simulink model "PMSM_Mathematical_Modeling"  (R2022a)
settings: Solver=VariableStepAuto  StartTime=0.0  StopTime=1  RelTol=1e-3
settings Model: Creator=nikos  LastModifiedBy=nikos

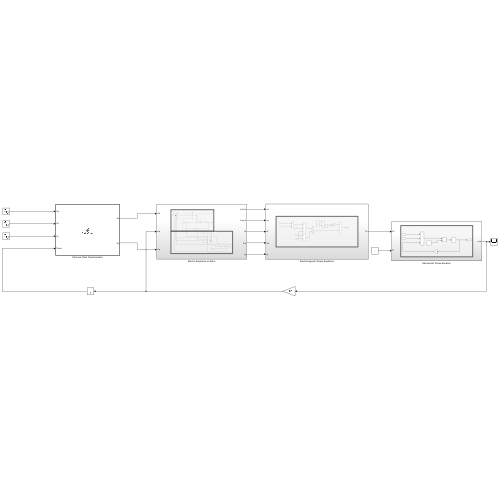
[thumbnail: Simulink's stored preview of the top-level diagram]
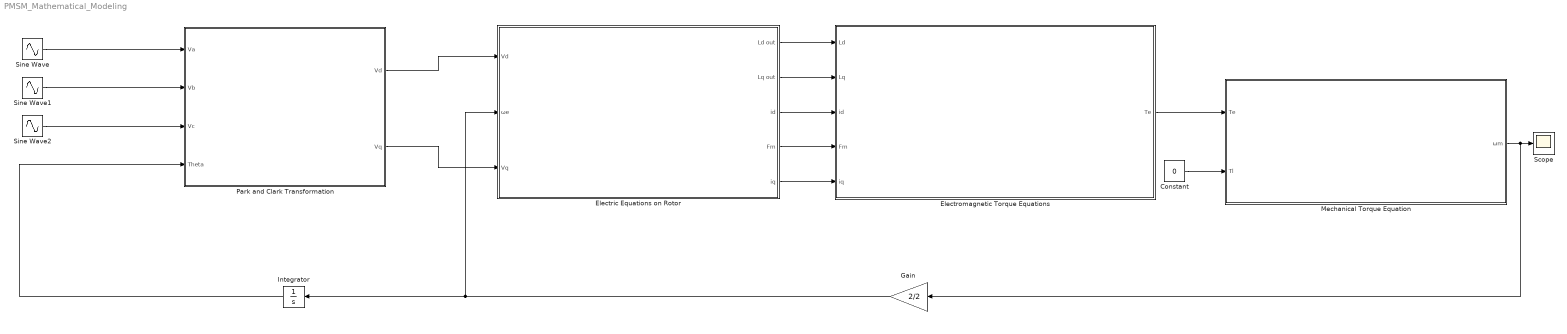
== system PMSM_Mathematical_Modeling ==
  Constant : Constant  Value=0
  Electric Equations on Rotor : Subsystem
  Electromagnetic Torque Equations : Subsystem
  Gain : Gain  Gain=2/2
  Integrator : Integrator
  Mechanical Torque Equation : Subsystem
  Park and Clark Transformation : MATLAB Function  TreatAsAtomicUnit=on
  Scope : Scope
  Sine Wave : Sin  Amplitude=240  Frequency=2*pi*50  SampleTime=0.001
  Sine Wave1 : Sin  Amplitude=240  Frequency=2*pi*50  Phase=-2*pi/3  SampleTime=0.001
  Sine Wave2 : Sin  Amplitude=240  Frequency=2*pi*50  Phase=2*pi/3  SampleTime=0.001
  wires:
  Park and Clark Transformation/1(Vd) -> Electric Equations on Rotor/1(Vd)
  Park and Clark Transformation/2(Vq) -> Electric Equations on Rotor/3(Vq)
  Electric Equations on Rotor/1(Ld out) -> Electromagnetic Torque Equations/1(Ld)
  Electric Equations on Rotor/2(Lq out) -> Electromagnetic Torque Equations/2(Lq)
  Electric Equations on Rotor/3(id) -> Electromagnetic Torque Equations/3(id)
  Electric Equations on Rotor/4(Fm) -> Electromagnetic Torque Equations/4(Fm)
  Electric Equations on Rotor/5(iq) -> Electromagnetic Torque Equations/5(iq)
  Electromagnetic Torque Equations/1(Te) -> Mechanical Torque Equation/1(Te)
  Constant/1 -> Mechanical Torque Equation/2(Tl)
  Mechanical Torque Equation/1(ωm) -> Scope/1, Gain/1
  Gain/1 -> Electric Equations on Rotor/2(ωe), Integrator/1
  Integrator/1 -> Park and Clark Transformation/4(Theta)
  Sine Wave2/1 -> Park and Clark Transformation/3(Vc)
  Sine Wave1/1 -> Park and Clark Transformation/2(Vb)
  Sine Wave/1 -> Park and Clark Transformation/1(Va)

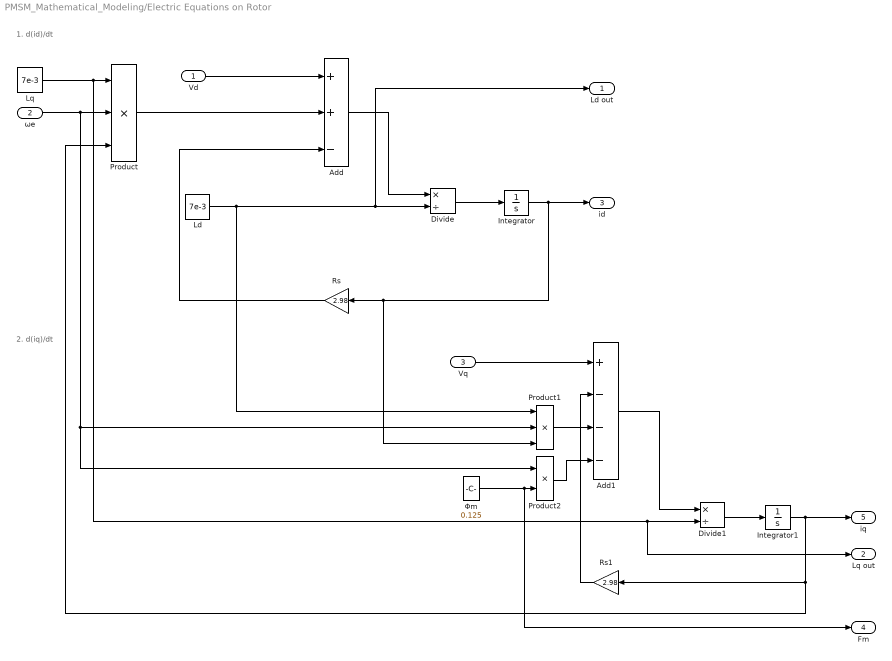
== system PMSM_Mathematical_Modeling/Electric Equations on Rotor ==
  note: 1. d(id)/dt
  note: 2. d(iq)/dt
  Vd : Inport
  ωe : Inport  Port=2
  Vq : Inport  Port=3
  Add : Sum  Inputs=++-
  Add1 : Sum  Inputs=+---
  Divide : Product  Inputs=*/
  Divide1 : Product  Inputs=*/
  Integrator : Integrator
  Integrator1 : Integrator
  Ld : Constant  Value=7e-3
  Lq : Constant  Value=7e-3
  Product : Product  Inputs=3
  Product1 : Product  Inputs=3
  Product2 : Product
  Rs : Gain  Gain=2.98
  Rs1 : Gain  Gain=2.98
  Φm : Constant  Value=0.125
  Ld out : Outport
  Lq out : Outport  Port=2
  id : Outport  Port=3
  Fm : Outport  Port=4
  iq : Outport  Port=5
  wires:
  Integrator1/1 -> iq/1, Product/3, Rs1/1
  Φm/1 -> Fm/1, Product2/2
  Lq/1 -> Lq out/1, Divide1/2, Product/1
  Integrator/1 -> id/1, Product1/3, Rs/1
  ωe/1 -> Product/2, Product2/1, Product1/2
  Ld/1 -> Product1/1, Ld out/1, Divide/2
  Rs/1 -> Add/3
  Vq/1 -> Add1/1
  Divide1/1 -> Integrator1/1
  Add1/1 -> Divide1/1
  Rs1/1 -> Add1/2
  Product1/1 -> Add1/3
  Product/1 -> Add/2
  Add/1 -> Divide/1
  Divide/1 -> Integrator/1
  Product2/1 -> Add1/4
  Vd/1 -> Add/1

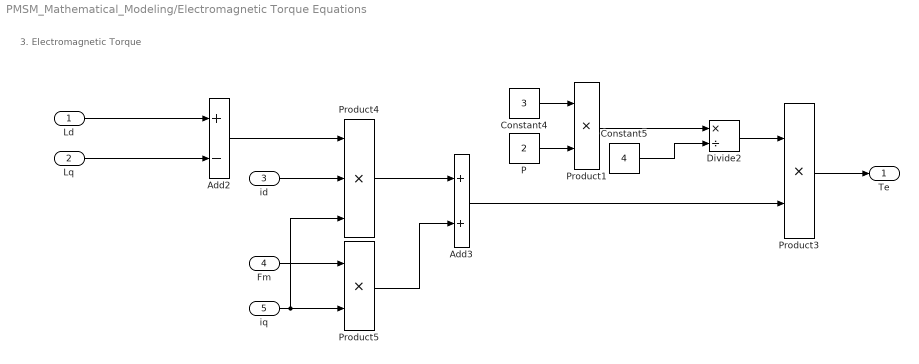
== system PMSM_Mathematical_Modeling/Electromagnetic Torque Equations ==
  note: 3. Electromagnetic Torque
  Ld : Inport
  Lq : Inport  Port=2
  id : Inport  Port=3
  Fm : Inport  Port=4
  iq : Inport  Port=5
  Add2 : Sum  Inputs=+-
  Add3 : Sum
  Constant4 : Constant  Value=3
  Constant5 : Constant  Value=4
  Divide2 : Product  Inputs=*/
  P : Constant  Value=2
  Product1 : Product
  Product3 : Product
  Product4 : Product  Inputs=3
  Product5 : Product
  Te : Outport
  wires:
  Product4/1 -> Add3/1
  Product5/1 -> Add3/2
  Add2/1 -> Product4/1
  iq/1 -> Product4/3, Product5/2
  Add3/1 -> Product3/2
  Lq/1 -> Add2/2
  id/1 -> Product4/2
  Ld/1 -> Add2/1
  Fm/1 -> Product5/1
  Constant4/1 -> Product1/1
  P/1 -> Product1/2
  Product1/1 -> Divide2/1
  Constant5/1 -> Divide2/2
  Divide2/1 -> Product3/1
  Product3/1 -> Te/1

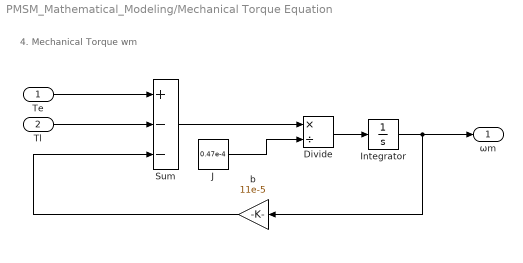
== system PMSM_Mathematical_Modeling/Mechanical Torque Equation ==
  note: 4. Mechanical Torque wm
  Te : Inport
  Tl : Inport  Port=2
  Divide : Product  Inputs=*/
  Integrator : Integrator
  J : Constant  Value=0.47e-4
  Sum : Sum  Inputs=+--
  b : Gain  Gain=11e-5
  ωm : Outport
  wires:
  Tl/1 -> Sum/2
  Divide/1 -> Integrator/1
  Sum/1 -> Divide/1
  Te/1 -> Sum/1
  J/1 -> Divide/2
  b/1 -> Sum/3
  Integrator/1 -> ωm/1, b/1

== matlab function PMSM_Mathematical_Modeling/Park and Clark Transformation ==
  data: Va input; Vd output; Vb input; Vc input; Theta input; Vq output
function [Vd, Vq] = ParknClark(Va, Vb, Vc, Theta)

if isempty(Theta)
    Theta = 0;
end

Vd = (2/3)*(Va*cos(Theta) + Vb*cos(Theta-(2*pi/3)) + Vc*cos(Theta + (2*pi/3)));
Vq = (2/3)*(-Va*sin(Theta) - Vb*sin(Theta-(2*pi/3)) - Vc*sin(Theta + (2*pi/3)));

end
